simulink library "lib_wheel2"  (Simulink 4.1.1)
values from neighbouring files (symbols this model uses):
  logFlag = 1    [advSACompMaskInit.m]    (also in advSACompMaskInitR13.m)
undefined symbols (not defined in the file or in its folder): lib_help, NOTES, veh_air_density, veh_CD, veh_cg_height, veh_FA, veh_front_wt_frac, veh_gravity, veh_roadwheel_radius, veh_rr_a, veh_rr_alpha, veh_rr_b, veh_rr_beta, veh_rr_c, veh_wheelbase, wh_1st_rrc, wh_2nd_rrc, wh_axle_loss_mass, wh_axle_loss_trq, wh_fa_dl_brake_frac, wh_fa_dl_brake_mph, wh_fa_fric_brake_frac, wh_fa_fric_brake_mph, wh_front_active_bool, wh_inertia, wh_max_front_brake_force, wh_max_rear_brake_force, wh_pressure, wh_radius, wh_rear_active_bool, wh_slip, wh_slip_force_coeff
libraries: lib_wheel2 x61, lib_vehicle x2, lib_etc x2, lib_controls x2, lib_wheel x1
(part 10 of 14)

== system lib_wheel2/vehicle, wheel, & axle front/rear <wh>/models and interface/wheel and axle  front/rear <wh>/limits and losses diagnostics ==
  speed : Inport  Orientation=down  Port=1  LatchInput=off
  front brake : Inport  Port=2  LatchInput=off
  front brake max : Inport  Port=3  LatchInput=off
  rear brake max : Inport  Port=4  LatchInput=off
  rear brake : Inport  Port=5  LatchInput=off
  Gain : Gain  Gain=-1  Multiplication=Element-wise(K.*u)  SaturateOnIntegerOverflow=on
  Logical Operator : Logic  Operator=OR  Inputs=2
  Product : Product  Inputs=2  Multiplication=Element-wise(.*)  SaturateOnIntegerOverflow=on
  Relational Operator1 : RelationalOperator  Operator===
  Relational Operator2 : RelationalOperator  Operator===
  Sum3 : Sum  Inputs=++  SaturateOnIntegerOverflow=on
  enhancedToWorkspace : Subsystem  TreatAsAtomicUnit=on  mask(enhancedToWorkspace){generalName=generalName01, specificName=brake_loss_pwr, logFlag=logFlag}
      mask prompts: generalName "General Name [char-evaluated]"; specificName "Specific Name [char-literal]"; logFlag "Enable flag (1=on,0=off)"
      mask help: A wrapper for the Simulink "To Workspace" block that allows you to evaluate the name of the variable to log to workspace. This is useful to avoid the double logging errors that occur when you pull in two library models that attempt to log to the same variable.
      mask init:
      | enhancedToWsMaker
      settings: CopyFcn=breakLinkCopyFcn  ParentCloseFcn=breakLinkParCloseFcn  RTWFcnNameOpts=Auto  RTWFileNameOpts=Auto
      mask Help:
      | <h2>Enhanced To Workspace Block</h2>
      | <h3>Parameters</h3>
      | <UL>
      | <li><b>General Name:</b> This is the more general name of the variable. Variables are saved to the workspace as <i>generalName_specificName</i>. Note that this is an evaluated variable. If you would like to type in the value directly, it must be surrounded with single quotes. Otherwise you can input the name of a variable containing a char string.</li>
      | <li><b>Specific Name:</b> This is the specific name of the variable. Note that this is input as a char literal (i.e., you don't need quotes).</li>
      | <li><b>Enable Flag:</b> This flag should have the value of 0 or 1. If 0, the variable will not be logged to the workspace. If 1, the variable will be logged. This is done so that variable logging can be turned off to improve speed.</li>
      | </ul>
      | <h3>Overview</h3>
      | <p>The enhanced to workspace block was put together to allow one to dynamically resolve variable names at run time in simulink. This is most powerful when used in conjunction with a masked subsystem to allow multiple instances of that masked subsytem to be used in the same model. The strategy is to set the generalName in the block mask which will allow the block to change the general name for all variable logging on the fly.
      | <h3>Helper Files</h3>
      | <p>Three m-files are required by the enhancedToWorkspace block. These files are located in the &lt; ADVISOR root &gt;/GUI directory :
      | <ul>
      | <li><i>enhancedToWsMaker.m</i> This file runs the mask initialization for the block</li>
      | <li><i>breakLinkCopyFcn.m</i> This file is used by the block callback when the simulink block is copied. It is necessary to break the link to the enhancedToWorkspace similar to the To Workspace block in order for it to be able to configure itself. (Try copying simulink's To Workspace block--it is impossible to make a link)</li>
      | <li><i>breakLinkParCloseFcn.m</i> This file is similar to the breakLinkCopyFcn and is used when a parent system is closed</li>
      | </ul>
      | <hr>
      | 
      | <p>Created 2003-Jan-21, Michael Patrick O'Keefe, NREL</p>
      | 
      | <!--
      | <VARDEF>
      | <H3>var_name</H3>
      | <UL>
      | <LI><B>data type</B> data type here</LI>
      | <LI><B>units</B> units here</LI>
      | <LI><B>vehicle type</B> vehicle type here</LI>
      | <LI><B>description</B> description here</LI>
      | </UL>
      | </VARDEF>
      | -->
      mask Display: disp([generalName,'_',specificName])
  tag scope: brake_limited=scoped
  wires:
  Gain/1 -> Product/2
  Sum3/1 -> Gain/1
  Product/1 -> enhancedToWorkspace/1(In1)
  Logical Operator/1 -> [brake_limited]
  Relational Operator1/1 -> Logical Operator/1
  Relational Operator2/1 -> Logical Operator/2
  speed/1 -> Product/1
  front brake/1 -> Sum3/1, Relational Operator1/1
  front brake max/1 -> Relational Operator1/2
  rear brake max/1 -> Relational Operator2/1
  rear brake/1 -> Sum3/2, Relational Operator2/2

== system lib_wheel2/vehicle, wheel, & axle front/rear <wh>/models and interface/wheel and axle  front/rear <wh>/loss (Nm) ==
  note: The loss torque is zero when the axle is not turning.
  axle speed (rad/s) : Inport  Port=1  LatchInput=off
  Constant : Constant  Orientation=up  Value=0
  Switch : Switch  Threshold=eps
  current veh mass : lib_wheel2/Submodels/current veh mass
      settings: RTWFcnNameOpts=Auto  RTWFileNameOpts=Auto
  wheel & axle bearing drag (Nm) : Lookup  InputValues=wh_axle_loss_mass  OutputValues=wh_axle_loss_trq
  drag torque (Nm) : Outport  Port=1  InitialOutput=0
  wires:
  current veh mass/1 -> wheel & axle bearing drag (Nm)/1
  Switch/1 -> drag torque (Nm)/1
  axle speed (rad/s)/1 -> Switch/2
  Constant/1 -> Switch/3
  wheel & axle bearing drag (Nm)/1 -> Switch/1

== system lib_wheel2/vehicle, wheel, & axle front/rear <wh>/models and interface/wheel and axle  front/rear <wh>/rear brake ==
  F_brake : Inport  Port=1  LatchInput=off
  Constant : Constant  Value=wh_max_rear_brake_force
  Terminator : Terminator
  F_brake_max : Outport  Port=1  InitialOutput=0
  wires:
  Constant/1 -> F_brake_max/1
  F_brake/1 -> Terminator/1

== system lib_wheel2/vehicle, wheel, & axle front/rear <wh>/models and interface/wheel and axle  front/rear <wh>/rear force ==
  In1 : Inport  Port=1  LatchInput=off
  In2 : Inport  Port=2  LatchInput=off
  Product2 : Product  Inputs=2  Multiplication=Element-wise(.*)  SaturateOnIntegerOverflow=on
  Sum1 : Sum  Inputs=-+  SaturateOnIntegerOverflow=on
  Sum4 : Sum  Inputs=-+  SaturateOnIntegerOverflow=on
  brake request controller interface1 : Subsystem
      settings: RTWFcnNameOpts=Auto  RTWFileNameOpts=Auto
  enhancedToWorkspace : Subsystem  TreatAsAtomicUnit=on  mask(enhancedToWorkspace){generalName=generalName01, specificName=rear_brake_r, logFlag=logFlag}
      mask prompts: generalName "General Name [char-evaluated]"; specificName "Specific Name [char-literal]"; logFlag "Enable flag (1=on,0=off)"
      mask help: A wrapper for the Simulink "To Workspace" block that allows you to evaluate the name of the variable to log to workspace. This is useful to avoid the double logging errors that occur when you pull in two library models that attempt to log to the same variable.
      mask init:
      | enhancedToWsMaker
      settings: CopyFcn=breakLinkCopyFcn  ParentCloseFcn=breakLinkParCloseFcn  RTWFcnNameOpts=Auto  RTWFileNameOpts=Auto
      mask Help:
      | <h2>Enhanced To Workspace Block</h2>
      | <h3>Parameters</h3>
      | <UL>
      | <li><b>General Name:</b> This is the more general name of the variable. Variables are saved to the workspace as <i>generalName_specificName</i>. Note that this is an evaluated variable. If you would like to type in the value directly, it must be surrounded with single quotes. Otherwise you can input the name of a variable containing a char string.</li>
      | <li><b>Specific Name:</b> This is the specific name of the variable. Note that this is input as a char literal (i.e., you don't need quotes).</li>
      | <li><b>Enable Flag:</b> This flag should have the value of 0 or 1. If 0, the variable will not be logged to the workspace. If 1, the variable will be logged. This is done so that variable logging can be turned off to improve speed.</li>
      | </ul>
      | <h3>Overview</h3>
      | <p>The enhanced to workspace block was put together to allow one to dynamically resolve variable names at run time in simulink. This is most powerful when used in conjunction with a masked subsystem to allow multiple instances of that masked subsytem to be used in the same model. The strategy is to set the generalName in the block mask which will allow the block to change the general name for all variable logging on the fly.
      | <h3>Helper Files</h3>
      | <p>Three m-files are required by the enhancedToWorkspace block. These files are located in the &lt; ADVISOR root &gt;/GUI directory :
      | <ul>
      | <li><i>enhancedToWsMaker.m</i> This file runs the mask initialization for the block</li>
      | <li><i>breakLinkCopyFcn.m</i> This file is used by the block callback when the simulink block is copied. It is necessary to break the link to the enhancedToWorkspace similar to the To Workspace block in order for it to be able to configure itself. (Try copying simulink's To Workspace block--it is impossible to make a link)</li>
      | <li><i>breakLinkParCloseFcn.m</i> This file is similar to the breakLinkCopyFcn and is used when a parent system is closed</li>
      | </ul>
      | <hr>
      | 
      | <p>Created 2003-Jan-21, Michael Patrick O'Keefe, NREL</p>
      | 
      | <!--
      | <VARDEF>
      | <H3>var_name</H3>
      | <UL>
      | <LI><B>data type</B> data type here</LI>
      | <LI><B>units</B> units here</LI>
      | <LI><B>vehicle type</B> vehicle type here</LI>
      | <LI><B>description</B> description here</LI>
      | </UL>
      | </VARDEF>
      | -->
      mask Display: disp([generalName,'_',specificName])
  tractive torque req/d of drivetrain (Nm)1 : Gain  Gain=wh_radius  Multiplication=Element-wise(K.*u)  SaturateOnIntegerOverflow=on
  Out1 : Outport  Port=1
  wires:
  brake request controller interface1/1(F_rear_brake_req) -> Sum4/1, enhancedToWorkspace/1(In1)
  Sum4/1 -> tractive torque req/d of drivetrain (Nm)1/1
  tractive torque req/d of drivetrain (Nm)1/1 -> Out1/1
  In1/1 -> Product2/1, Sum1/2
  In2/1 -> Product2/2
  Product2/1 -> Sum1/1
  Sum1/1 -> Sum4/2

== system lib_wheel2/vehicle, wheel, & axle front/rear <wh>/models and interface/wheel and axle  front/rear <wh>/tire slip model (m/s) ==
  note: See note regarding sum in backward path
  weight borne  by front axle (N) : Inport  Port=1  LatchInput=off
  total tractive  force available (N) : Inport  Port=2  LatchInput=off
  axle speed available (rad/s) : Inport  Port=3  LatchInput=off
  axle speed req'd (rad/s) : Inport  Port=4  LatchInput=off
  vehicle speed required (m/s) : Inport  Port=5  LatchInput=off
  weight borne by  rear axle (N) : Inport  Port=6  LatchInput=off
  front fraction : Inport  Port=7  LatchInput=off
  Abs1 : Abs  SaturateOnIntegerOverflow=on
  Block NOTES : Subsystem
      settings: RTWFcnNameOpts=Auto  RTWFileNameOpts=Auto
      mask Display: disp('Block\nNOTES')
  Constant : Constant  Orientation=left  Value=1e-3
  Constant5 : Constant  Value=1
  Constant6 : Constant  Orientation=left  Value=wh_radius
  Fcn : Fcn  Expr=1/u
  Relational Operator1 : RelationalOperator  Operator=>
  Sum1 : Sum  Inputs=+-  SaturateOnIntegerOverflow=on
  Sum2 : Sum  Inputs=++  SaturateOnIntegerOverflow=on
  Sum3 : Sum  Inputs=++  SaturateOnIntegerOverflow=on
  Sum4 : Sum  Inputs=-+  SaturateOnIntegerOverflow=on
  Switch1 : Switch  Threshold=eps
  front axle : Subsystem
      settings: RTWFcnNameOpts=Auto  RTWFileNameOpts=Auto
  front frac : Product  Inputs=2  Multiplication=Element-wise(.*)  SaturateOnIntegerOverflow=on
  rear axle : Subsystem
      settings: RTWFcnNameOpts=Auto  RTWFileNameOpts=Auto
  vehicle speed (m/s) : Product  Inputs=3  Multiplication=Element-wise(.*)  SaturateOnIntegerOverflow=on
  possible vehicle speed (m/s) : Outport  Port=1  InitialOutput=0
  tag scope: veh_spd_a_rec=scoped
  wires:
  Sum3/1 -> Fcn/1
  Fcn/1 -> vehicle speed (m/s)/1
  Constant5/1 -> Sum3/2
  axle speed available (rad/s)/1 -> Sum4/1, vehicle speed (m/s)/2
  Constant6/1 -> vehicle speed (m/s)/3
  Relational Operator1/1 -> Switch1/2
  vehicle speed required (m/s)/1 -> Switch1/3
  Sum4/1 -> Abs1/1
  axle speed req'd (rad/s)/1 -> Sum4/2
  Constant/1 -> Relational Operator1/2
  Abs1/1 -> Relational Operator1/1
  weight borne  by front axle (N)/1 -> front axle/1(In1)
  Switch1/1 -> possible vehicle speed (m/s)/1
  vehicle speed (m/s)/1 -> Switch1/1, [veh_spd_a_rec]
  weight borne by  rear axle (N)/1 -> rear axle/1(In1)
  total tractive  force available (N)/1 -> front frac/1, Sum1/1
  front fraction/1 -> front frac/2
  front frac/1 -> front axle/2(In2), Sum1/2
  Sum1/1 -> rear axle/2(In2)
  front axle/1(Out1) -> Sum2/1
  rear axle/1(Out1) -> Sum2/2
  Sum2/1 -> Sum3/1

== system lib_wheel2/vehicle, wheel, & axle front/rear <wh>/models and interface/wheel and axle  front/rear <wh>/tire slip model (rad/s) ==
  note: Slip is defined as s=(omega*r - v) / v.  The one-to-one mapping of slip to normalized
      | tractive force, F_tract/W_front_axle, up to the maximum, is stored in the variables
      | "wh_slip" and "wh_slip_force_coeff."
  note: This block implements the effects of finite tire slip
      | (with respect to the road) on the vehicle speed/wheel speed relationship.
  note: Question: for front and rear, is it the sum of or min/max? tm:020703
  total tractive  force requested (N) : Inport  Port=1  LatchInput=off
  requested time-step average vehicle speed (m/s) : Inport  Port=2  LatchInput=off
  weight borne by front axle (N) : Inport  Port=3  LatchInput=off
  weight borne by  rear axle (N)1 : Inport  Port=4  LatchInput=off
  front traction ratio : Inport  Port=5  LatchInput=off
  Constant5 : Constant  Value=1
  Constant6 : Constant  Orientation=up  Value=1/wh_radius
  Sum1 : Sum  Inputs=+-  SaturateOnIntegerOverflow=on
  Sum2 : Sum  Inputs=++  SaturateOnIntegerOverflow=on
  Sum3 : Sum  Inputs=++  SaturateOnIntegerOverflow=on
  enhancedToWorkspace : Subsystem  TreatAsAtomicUnit=on  mask(enhancedToWorkspace){generalName=generalName01, specificName=slip_r, logFlag=logFlag}
      mask prompts: generalName "General Name [char-evaluated]"; specificName "Specific Name [char-literal]"; logFlag "Enable flag (1=on,0=off)"
      mask help: A wrapper for the Simulink "To Workspace" block that allows you to evaluate the name of the variable to log to workspace. This is useful to avoid the double logging errors that occur when you pull in two library models that attempt to log to the same variable.
      mask init:
      | enhancedToWsMaker
      settings: CopyFcn=breakLinkCopyFcn  ParentCloseFcn=breakLinkParCloseFcn  RTWFcnNameOpts=Auto  RTWFileNameOpts=Auto
      mask Help:
      | <h2>Enhanced To Workspace Block</h2>
      | <h3>Parameters</h3>
      | <UL>
      | <li><b>General Name:</b> This is the more general name of the variable. Variables are saved to the workspace as <i>generalName_specificName</i>. Note that this is an evaluated variable. If you would like to type in the value directly, it must be surrounded with single quotes. Otherwise you can input the name of a variable containing a char string.</li>
      | <li><b>Specific Name:</b> This is the specific name of the variable. Note that this is input as a char literal (i.e., you don't need quotes).</li>
      | <li><b>Enable Flag:</b> This flag should have the value of 0 or 1. If 0, the variable will not be logged to the workspace. If 1, the variable will be logged. This is done so that variable logging can be turned off to improve speed.</li>
      | </ul>
      | <h3>Overview</h3>
      | <p>The enhanced to workspace block was put together to allow one to dynamically resolve variable names at run time in simulink. This is most powerful when used in conjunction with a masked subsystem to allow multiple instances of that masked subsytem to be used in the same model. The strategy is to set the generalName in the block mask which will allow the block to change the general name for all variable logging on the fly.
      | <h3>Helper Files</h3>
      | <p>Three m-files are required by the enhancedToWorkspace block. These files are located in the &lt; ADVISOR root &gt;/GUI directory :
      | <ul>
      | <li><i>enhancedToWsMaker.m</i> This file runs the mask initialization for the block</li>
      | <li><i>breakLinkCopyFcn.m</i> This file is used by the block callback when the simulink block is copied. It is necessary to break the link to the enhancedToWorkspace similar to the To Workspace block in order for it to be able to configure itself. (Try copying simulink's To Workspace block--it is impossible to make a link)</li>
      | <li><i>breakLinkParCloseFcn.m</i> This file is similar to the breakLinkCopyFcn and is used when a parent system is closed</li>
      | </ul>
      | <hr>
      | 
      | <p>Created 2003-Jan-21, Michael Patrick O'Keefe, NREL</p>
      | 
      | <!--
      | <VARDEF>
      | <H3>var_name</H3>
      | <UL>
      | <LI><B>data type</B> data type here</LI>
      | <LI><B>units</B> units here</LI>
      | <LI><B>vehicle type</B> vehicle type here</LI>
      | <LI><B>description</B> description here</LI>
      | </UL>
      | </VARDEF>
      | -->
      mask Display: disp([generalName,'_',specificName])
  front frac : Product  Inputs=2  Multiplication=Element-wise(.*)  SaturateOnIntegerOverflow=on
  front slip : Subsystem
      settings: RTWFcnNameOpts=Auto  RTWFileNameOpts=Auto
  rear slip : Subsystem
      settings: RTWFcnNameOpts=Auto  RTWFileNameOpts=Auto
  wheel speed (rad/s) : Product  Inputs=3  Multiplication=Element-wise(.*)  SaturateOnIntegerOverflow=on
  slip-augmented rotational speed (rad/s) : Outport  Port=1  InitialOutput=0
  wires:
  weight borne by front axle (N)/1 -> front slip/1(In1)
  requested time-step average vehicle speed (m/s)/1 -> wheel speed (rad/s)/1
  Constant6/1 -> wheel speed (rad/s)/3
  Sum3/1 -> wheel speed (rad/s)/2
  Constant5/1 -> Sum3/2
  wheel speed (rad/s)/1 -> slip-augmented rotational speed (rad/s)/1
  front frac/1 -> Sum1/2, front slip/2(In2)
  total tractive  force requested (N)/1 -> front frac/1, Sum1/1
  front traction ratio/1 -> front frac/2
  Sum1/1 -> rear slip/2(In2)
  weight borne by  rear axle (N)1/1 -> rear slip/1(In1)
  front slip/1(Out1) -> Sum2/1
  rear slip/1(Out1) -> Sum2/2
  Sum2/1 -> Sum3/1, enhancedToWorkspace/1(In1)

== system lib_wheel2/vehicle, wheel, & axle front/rear <wh>/models and interface/wheel and axle  front/rear <wh>/traction controller interface ==
  F_req : Inport  Port=1  LatchInput=off
  v_ave_req : Inport  Port=2  LatchInput=off
  F_req_limited : Outport  Port=1  InitialOutput=0
  v_req_limited : Outport  Port=2  InitialOutput=0
  wt_front_axle : Outport  Port=3  InitialOutput=0
  wt_rear_axle : Outport  Port=4  InitialOutput=0
  front_traction_ratio : Outport  Port=5  InitialOutput=0
  tag scope: F_req=scoped, v_ave_req=scoped
  wires:
  [F_req_limited] -> F_req_limited/1
  [v_req_limited] -> v_req_limited/1
  [wt_front_axle] -> wt_front_axle/1
  F_req/1 -> [F_req]
  v_ave_req/1 -> [v_ave_req]
  [wt_rear_axle] -> wt_rear_axle/1
  [front_traction_ratio] -> front_traction_ratio/1

== system lib_wheel2/vehicle, wheel, & axle front/rear <wh> 2 axle --> 1 driveline/models and interface/vehicle <veh>/Block NOTES ==
  note: Given the tractive force available, this block uses the same equations to determine the achievable speed.
  note: If no drivetrain component ran up against its performance limit during the time step, the achieved speed
      | is taken to be the requested speed.
  note: This block uses the required vehicle speed with vehicle parameters and the previous speed
      | and classic, straightforward equations to determine the tractive force required at the tire/road interface.
  note: A slight simplification, the assumption that (speed_at_end_of_time_step)^2 is roughly equal to
      | (speed_at_end_of_time_step)*(speed_at_beginning_of_time_step), is used to avoid solving
      | a quadratic equation in the solution of v=v(Ftract).
  note: 2003-April-02, Michael O'Keefe
      | Model updated to use a "stand-alone" mask format

== system lib_wheel2/vehicle, wheel, & axle front/rear <wh> 2 axle --> 1 driveline/models and interface/vehicle <veh>/enhancedToWorkspace ==
  In1 : Inport  Port=1  LatchInput=off
  To Workspace : ToWorkspace  VariableName=veh_spd_a  SampleTime=-1  SaveFormat=Array
  wires:
  In1/1 -> To Workspace/1

== system lib_wheel2/vehicle, wheel, & axle front/rear <wh> 2 axle --> 1 driveline/models and interface/vehicle <veh>/enhancedToWorkspace1 ==
  In1 : Inport  Port=1  LatchInput=off
  To Workspace : ToWorkspace  VariableName=veh_force_a  SampleTime=-1  SaveFormat=Array
  wires:
  In1/1 -> To Workspace/1

== system lib_wheel2/vehicle, wheel, & axle front/rear <wh> 2 axle --> 1 driveline/models and interface/vehicle <veh>/enhancedToWorkspace2 ==
  In1 : Inport  Port=1  LatchInput=off
  To Workspace : ToWorkspace  VariableName=veh_spd_r  SampleTime=-1  SaveFormat=Array
  wires:
  In1/1 -> To Workspace/1

== system lib_wheel2/vehicle, wheel, & axle front/rear <wh> 2 axle --> 1 driveline/models and interface/vehicle <veh>/enhancedToWorkspace3 ==
  In1 : Inport  Port=1  LatchInput=off
  To Workspace : ToWorkspace  VariableName=veh_force_r  SampleTime=-1  SaveFormat=Array
  wires:
  In1/1 -> To Workspace/1

== system lib_wheel2/vehicle, wheel, & axle front/rear <wh> 2 axle --> 1 driveline/models and interface/vehicle <veh>/enhancedToWorkspace4 ==
  In1 : Inport  Port=1  LatchInput=off
  To Workspace : ToWorkspace  VariableName=veh_Fr  SampleTime=-1  SaveFormat=Array
  wires:
  In1/1 -> To Workspace/1

== system lib_wheel2/vehicle, wheel, & axle front/rear <wh> 2 axle --> 1 driveline/models and interface/vehicle <veh>/force req'd to accelerate (N) ==
  v(m/s) : Inport  Port=1  LatchInput=off
  v prev : Inport  Port=2  LatchInput=off
  Clock : Clock
      settings: DisplayTime=off  Decimation=10
  Memory : Memory  X0=-0.1  InheritSampleTime=off
      settings: RTWStateStorageClass=Auto
  Product1 : Product  Inputs=**/  Multiplication=Element-wise(.*)  SaturateOnIntegerOverflow=on
  Sum : Sum  Inputs=+-  SaturateOnIntegerOverflow=on
  Sum1 : Sum  Inputs=+-  SaturateOnIntegerOverflow=on
  current veh mass : lib_wheel2/Submodels/current veh mass
      settings: RTWFcnNameOpts=Auto  RTWFileNameOpts=Auto
  (N) : Outport  Port=1  InitialOutput=0
  wires:
  Sum/1 -> Product1/2
  Sum1/1 -> Product1/3
  v(m/s)/1 -> Sum/1
  v prev/1 -> Sum/2
  Product1/1 -> (N)/1
  Memory/1 -> Sum1/2
  Clock/1 -> Memory/1, Sum1/1
  current veh mass/1 -> Product1/1

== system lib_wheel2/vehicle, wheel, & axle front/rear <wh> 2 axle --> 1 driveline/models and interface/vehicle <veh>/force req'd to ascend (N) ==
  average vehicle speed over time step (m/s) : Inport  Port=1  LatchInput=off
  Constant : Constant  Value=veh_gravity
  Constant1 : Constant  Value=0
  Product : Product  Inputs=3  Multiplication=Element-wise(.*)  SaturateOnIntegerOverflow=on
  Switch : Switch  Threshold=0
  Trigonometric Function : Trigonometry  Operator=atan  OutputSignalType=auto
  Trigonometric Function1 : Trigonometry  Operator=sin  OutputSignalType=auto
  current veh mass : lib_wheel2/Submodels/current veh mass
      settings: RTWFcnNameOpts=Auto  RTWFileNameOpts=Auto
  (N) : Outport  Port=1  InitialOutput=0
  wires:
  Trigonometric Function/1 -> Trigonometric Function1/1
  Trigonometric Function1/1 -> Product/2
  [grade] -> Trigonometric Function/1
  Constant/1 -> Product/1
  Product/1 -> Switch/1
  Switch/1 -> (N)/1
  Constant1/1 -> Switch/3
  average vehicle speed over time step (m/s)/1 -> Switch/2
  current veh mass/1 -> Product/3

== system lib_wheel2/vehicle, wheel, & axle front/rear <wh> 2 axle --> 1 driveline/models and interface/vehicle <veh>/force req'd to overcome aerodynamic drag (N) ==
  average vehicle speed over time step (m/s) : Inport  Port=1  LatchInput=off
  Constant : Constant  Value=veh_air_density*veh_CD*veh_FA*0.5
  Product : Product  Inputs=3  Multiplication=Element-wise(.*)  SaturateOnIntegerOverflow=on
  D aero(N) : Outport  Port=1  InitialOutput=0
  wires:
  average vehicle speed over time step (m/s)/1 -> Product/1, Product/2
  Constant/1 -> Product/3
  Product/1 -> D aero(N)/1

== system lib_wheel2/vehicle, wheel, & axle front/rear <wh> 2 axle --> 1 driveline/models and interface/vehicle <veh>/help ==

== system lib_wheel2/vehicle, wheel, & axle front/rear <wh> 2 axle --> 1 driveline/models and interface/vehicle <veh>/memory & init speed ==
  note: cyc_mph(1,2)*.447
  note: 2003-April-02, Michael O'Keefe
      |
      | This block passes through the last speed achieved unless this is the initial condition in which
      | case the initial speed value (a supplied control signal) is passed through. For backwards
      | compatibility, the value of v_init should be cyc_mph(1,2)*0.447
  signal in : Inport  Port=1  LatchInput=off
  signal init : Inport  Port=2  LatchInput=off
  Constant : Constant  Value=1
  IC : InitialCondition  Value=0
  Memory : Memory  X0=0  InheritSampleTime=off
      settings: RTWStateStorageClass=Auto
  Switch : Switch  Threshold=0.5
  signal out : Outport  Port=1
  wires:
  signal in/1 -> Memory/1
  Constant/1 -> IC/1
  Memory/1 -> Switch/1
  IC/1 -> Switch/2
  Switch/1 -> signal out/1
  signal init/1 -> Switch/3

== system lib_wheel2/vehicle, wheel, & axle front/rear <wh> 2 axle --> 1 driveline/models and interface/vehicle <veh>/power logging--achieved ==
  veh_force_a : Inport  Port=1  LatchInput=off
  veh_spd_a : Inport  Port=2  LatchInput=off
  Integrator : Integrator  ExternalReset=none  InitialConditionSource=internal  InitialCondition=0  LimitOutput=off  UpperSaturationLimit=inf  LowerSaturationLimit=-inf  ShowSaturationPort=off  ShowStatePort=off  AbsoluteTolerance=auto
  Joules : Subsystem  TreatAsAtomicUnit=on  mask(enhancedToWorkspace){generalName=generalName, specificName=energy_a, logFlag=logFlag}
      mask prompts: generalName "General Name [char-evaluated]"; specificName "Specific Name [char-literal]"; logFlag "Enable flag (1=on,0=off)"
      mask help: A wrapper for the Simulink "To Workspace" block that allows you to evaluate the name of the variable to log to workspace. This is useful to avoid the double logging errors that occur when you pull in two library models that attempt to log to the same variable.
      mask init:
      | enhancedToWsMaker
      settings: CopyFcn=breakLinkCopyFcn  ParentCloseFcn=breakLinkParCloseFcn  RTWFcnNameOpts=Auto  RTWFileNameOpts=Auto
      mask Help:
      | <h2>Enhanced To Workspace Block</h2>
      | <h3>Parameters</h3>
      | <UL>
      | <li><b>General Name:</b> This is the more general name of the variable. Variables are saved to the workspace as <i>generalName_specificName</i>. Note that this is an evaluated variable. If you would like to type in the value directly, it must be surrounded with single quotes. Otherwise you can input the name of a variable containing a char string.</li>
      | <li><b>Specific Name:</b> This is the specific name of the variable. Note that this is input as a char literal (i.e., you don't need quotes).</li>
      | <li><b>Enable Flag:</b> This flag should have the value of 0 or 1. If 0, the variable will not be logged to the workspace. If 1, the variable will be logged. This is done so that variable logging can be turned off to improve speed.</li>
      | </ul>
      | <h3>Overview</h3>
      | <p>The enhanced to workspace block was put together to allow one to dynamically resolve variable names at run time in simulink. This is most powerful when used in conjunction with a masked subsystem to allow multiple instances of that masked subsytem to be used in the same model. The strategy is to set the generalName in the block mask which will allow the block to change the general name for all variable logging on the fly.
      | <h3>Helper Files</h3>
      | <p>Three m-files are required by the enhancedToWorkspace block. These files are located in the &lt; ADVISOR root &gt;/GUI directory :
      | <ul>
      | <li><i>enhancedToWsMaker.m</i> This file runs the mask initialization for the block</li>
      | <li><i>breakLinkCopyFcn.m</i> This file is used by the block callback when the simulink block is copied. It is necessary to break the link to the enhancedToWorkspace similar to the To Workspace block in order for it to be able to configure itself. (Try copying simulink's To Workspace block--it is impossible to make a link)</li>
      | <li><i>breakLinkParCloseFcn.m</i> This file is similar to the breakLinkCopyFcn and is used when a parent system is closed</li>
      | </ul>
      | <hr>
      | 
      | <p>Created 2003-Jan-21, Michael Patrick O'Keefe, NREL</p>
      | 
      | <!--
      | <VARDEF>
      | <H3>var_name</H3>
      | <UL>
      | <LI><B>data type</B> data type here</LI>
      | <LI><B>units</B> units here</LI>
      | <LI><B>vehicle type</B> vehicle type here</LI>
      | <LI><B>description</B> description here</LI>
      | </UL>
      | </VARDEF>
      | -->
      mask Display: disp([generalName,'_',specificName])
  Product : Product  Inputs=2  Multiplication=Element-wise(.*)  SaturateOnIntegerOverflow=on
  horse power : Subsystem  TreatAsAtomicUnit=on  mask(enhancedToWorkspace){generalName=generalName, specificName=pwr_a_hp, logFlag=logFlag}
      mask prompts: generalName "General Name [char-evaluated]"; specificName "Specific Name [char-literal]"; logFlag "Enable flag (1=on,0=off)"
      mask help: A wrapper for the Simulink "To Workspace" block that allows you to evaluate the name of the variable to log to workspace. This is useful to avoid the double logging errors that occur when you pull in two library models that attempt to log to the same variable.
      mask init:
      | enhancedToWsMaker
      settings: CopyFcn=breakLinkCopyFcn  ParentCloseFcn=breakLinkParCloseFcn  RTWFcnNameOpts=Auto  RTWFileNameOpts=Auto
      mask Help:
      | <h2>Enhanced To Workspace Block</h2>
      | <h3>Parameters</h3>
      | <UL>
      | <li><b>General Name:</b> This is the more general name of the variable. Variables are saved to the workspace as <i>generalName_specificName</i>. Note that this is an evaluated variable. If you would like to type in the value directly, it must be surrounded with single quotes. Otherwise you can input the name of a variable containing a char string.</li>
      | <li><b>Specific Name:</b> This is the specific name of the variable. Note that this is input as a char literal (i.e., you don't need quotes).</li>
      | <li><b>Enable Flag:</b> This flag should have the value of 0 or 1. If 0, the variable will not be logged to the workspace. If 1, the variable will be logged. This is done so that variable logging can be turned off to improve speed.</li>
      | </ul>
      | <h3>Overview</h3>
      | <p>The enhanced to workspace block was put together to allow one to dynamically resolve variable names at run time in simulink. This is most powerful when used in conjunction with a masked subsystem to allow multiple instances of that masked subsytem to be used in the same model. The strategy is to set the generalName in the block mask which will allow the block to change the general name for all variable logging on the fly.
      | <h3>Helper Files</h3>
      | <p>Three m-files are required by the enhancedToWorkspace block. These files are located in the &lt; ADVISOR root &gt;/GUI directory :
      | <ul>
      | <li><i>enhancedToWsMaker.m</i> This file runs the mask initialization for the block</li>
      | <li><i>breakLinkCopyFcn.m</i> This file is used by the block callback when the simulink block is copied. It is necessary to break the link to the enhancedToWorkspace similar to the To Workspace block in order for it to be able to configure itself. (Try copying simulink's To Workspace block--it is impossible to make a link)</li>
      | <li><i>breakLinkParCloseFcn.m</i> This file is similar to the breakLinkCopyFcn and is used when a parent system is closed</li>
      | </ul>
      | <hr>
      | 
      | <p>Created 2003-Jan-21, Michael Patrick O'Keefe, NREL</p>
      | 
      | <!--
      | <VARDEF>
      | <H3>var_name</H3>
      | <UL>
      | <LI><B>data type</B> data type here</LI>
      | <LI><B>units</B> units here</LI>
      | <LI><B>vehicle type</B> vehicle type here</LI>
      | <LI><B>description</B> description here</LI>
      | </UL>
      | </VARDEF>
      | -->
      mask Display: disp([generalName,'_',specificName])
  "w -> hp" : Gain  Gain=0.001341022  Multiplication=Element-wise(K.*u)  SaturateOnIntegerOverflow=on
  watts : Subsystem  TreatAsAtomicUnit=on  mask(enhancedToWorkspace){generalName=generalName, specificName=pwr_a, logFlag=logFlag}
      mask prompts: generalName "General Name [char-evaluated]"; specificName "Specific Name [char-literal]"; logFlag "Enable flag (1=on,0=off)"
      mask help: A wrapper for the Simulink "To Workspace" block that allows you to evaluate the name of the variable to log to workspace. This is useful to avoid the double logging errors that occur when you pull in two library models that attempt to log to the same variable.
      mask init:
      | enhancedToWsMaker
      settings: CopyFcn=breakLinkCopyFcn  ParentCloseFcn=breakLinkParCloseFcn  RTWFcnNameOpts=Auto  RTWFileNameOpts=Auto
      mask Help:
      | <h2>Enhanced To Workspace Block</h2>
      | <h3>Parameters</h3>
      | <UL>
      | <li><b>General Name:</b> This is the more general name of the variable. Variables are saved to the workspace as <i>generalName_specificName</i>. Note that this is an evaluated variable. If you would like to type in the value directly, it must be surrounded with single quotes. Otherwise you can input the name of a variable containing a char string.</li>
      | <li><b>Specific Name:</b> This is the specific name of the variable. Note that this is input as a char literal (i.e., you don't need quotes).</li>
      | <li><b>Enable Flag:</b> This flag should have the value of 0 or 1. If 0, the variable will not be logged to the workspace. If 1, the variable will be logged. This is done so that variable logging can be turned off to improve speed.</li>
      | </ul>
      | <h3>Overview</h3>
      | <p>The enhanced to workspace block was put together to allow one to dynamically resolve variable names at run time in simulink. This is most powerful when used in conjunction with a masked subsystem to allow multiple instances of that masked subsytem to be used in the same model. The strategy is to set the generalName in the block mask which will allow the block to change the general name for all variable logging on the fly.
      | <h3>Helper Files</h3>
      | <p>Three m-files are required by the enhancedToWorkspace block. These files are located in the &lt; ADVISOR root &gt;/GUI directory :
      | <ul>
      | <li><i>enhancedToWsMaker.m</i> This file runs the mask initialization for the block</li>
      | <li><i>breakLinkCopyFcn.m</i> This file is used by the block callback when the simulink block is copied. It is necessary to break the link to the enhancedToWorkspace similar to the To Workspace block in order for it to be able to configure itself. (Try copying simulink's To Workspace block--it is impossible to make a link)</li>
      | <li><i>breakLinkParCloseFcn.m</i> This file is similar to the breakLinkCopyFcn and is used when a parent system is closed</li>
      | </ul>
      | <hr>
      | 
      | <p>Created 2003-Jan-21, Michael Patrick O'Keefe, NREL</p>
      | 
      | <!--
      | <VARDEF>
      | <H3>var_name</H3>
      | <UL>
      | <LI><B>data type</B> data type here</LI>
      | <LI><B>units</B> units here</LI>
      | <LI><B>vehicle type</B> vehicle type here</LI>
      | <LI><B>description</B> description here</LI>
      | </UL>
      | </VARDEF>
      | -->
      mask Display: disp([generalName,'_',specificName])
  wires:
  veh_spd_a/1 -> Product/2
  veh_force_a/1 -> Product/1
  Integrator/1 -> Joules/1(In1)
  Product/1 -> watts/1(In1), Integrator/1, "w -> hp"/1
  "w -> hp"/1 -> horse power/1(In1)

== system lib_wheel2/vehicle, wheel, & axle front/rear <wh> 2 axle --> 1 driveline/models and interface/vehicle <veh>/power logging--request ==
  veh_force_r : Inport  Port=1  LatchInput=off
  veh_spd_r : Inport  Port=2  LatchInput=off
  Integrator : Integrator  ExternalReset=none  InitialConditionSource=internal  InitialCondition=0  LimitOutput=off  UpperSaturationLimit=inf  LowerSaturationLimit=-inf  ShowSaturationPort=off  ShowStatePort=off  AbsoluteTolerance=auto
  Joules : Subsystem  TreatAsAtomicUnit=on  mask(enhancedToWorkspace){generalName=generalName, specificName=energy_r, logFlag=logFlag}
      mask prompts: generalName "General Name [char-evaluated]"; specificName "Specific Name [char-literal]"; logFlag "Enable flag (1=on,0=off)"
      mask help: A wrapper for the Simulink "To Workspace" block that allows you to evaluate the name of the variable to log to workspace. This is useful to avoid the double logging errors that occur when you pull in two library models that attempt to log to the same variable.
      mask init:
      | enhancedToWsMaker
      settings: CopyFcn=breakLinkCopyFcn  ParentCloseFcn=breakLinkParCloseFcn  RTWFcnNameOpts=Auto  RTWFileNameOpts=Auto
      mask Help:
      | <h2>Enhanced To Workspace Block</h2>
      | <h3>Parameters</h3>
      | <UL>
      | <li><b>General Name:</b> This is the more general name of the variable. Variables are saved to the workspace as <i>generalName_specificName</i>. Note that this is an evaluated variable. If you would like to type in the value directly, it must be surrounded with single quotes. Otherwise you can input the name of a variable containing a char string.</li>
      | <li><b>Specific Name:</b> This is the specific name of the variable. Note that this is input as a char literal (i.e., you don't need quotes).</li>
      | <li><b>Enable Flag:</b> This flag should have the value of 0 or 1. If 0, the variable will not be logged to the workspace. If 1, the variable will be logged. This is done so that variable logging can be turned off to improve speed.</li>
      | </ul>
      | <h3>Overview</h3>
      | <p>The enhanced to workspace block was put together to allow one to dynamically resolve variable names at run time in simulink. This is most powerful when used in conjunction with a masked subsystem to allow multiple instances of that masked subsytem to be used in the same model. The strategy is to set the generalName in the block mask which will allow the block to change the general name for all variable logging on the fly.
      | <h3>Helper Files</h3>
      | <p>Three m-files are required by the enhancedToWorkspace block. These files are located in the &lt; ADVISOR root &gt;/GUI directory :
      | <ul>
      | <li><i>enhancedToWsMaker.m</i> This file runs the mask initialization for the block</li>
      | <li><i>breakLinkCopyFcn.m</i> This file is used by the block callback when the simulink block is copied. It is necessary to break the link to the enhancedToWorkspace similar to the To Workspace block in order for it to be able to configure itself. (Try copying simulink's To Workspace block--it is impossible to make a link)</li>
      | <li><i>breakLinkParCloseFcn.m</i> This file is similar to the breakLinkCopyFcn and is used when a parent system is closed</li>
      | </ul>
      | <hr>
      | 
      | <p>Created 2003-Jan-21, Michael Patrick O'Keefe, NREL</p>
      | 
      | <!--
      | <VARDEF>
      | <H3>var_name</H3>
      | <UL>
      | <LI><B>data type</B> data type here</LI>
      | <LI><B>units</B> units here</LI>
      | <LI><B>vehicle type</B> vehicle type here</LI>
      | <LI><B>description</B> description here</LI>
      | </UL>
      | </VARDEF>
      | -->
      mask Display: disp([generalName,'_',specificName])
  Product : Product  Inputs=2  Multiplication=Element-wise(.*)  SaturateOnIntegerOverflow=on
  horse power : Subsystem  TreatAsAtomicUnit=on  mask(enhancedToWorkspace){generalName=generalName, specificName=pwr_r_hp, logFlag=logFlag}
      mask prompts: generalName "General Name [char-evaluated]"; specificName "Specific Name [char-literal]"; logFlag "Enable flag (1=on,0=off)"
      mask help: A wrapper for the Simulink "To Workspace" block that allows you to evaluate the name of the variable to log to workspace. This is useful to avoid the double logging errors that occur when you pull in two library models that attempt to log to the same variable.
      mask init:
      | enhancedToWsMaker
      settings: CopyFcn=breakLinkCopyFcn  ParentCloseFcn=breakLinkParCloseFcn  RTWFcnNameOpts=Auto  RTWFileNameOpts=Auto
      mask Help:
      | <h2>Enhanced To Workspace Block</h2>
      | <h3>Parameters</h3>
      | <UL>
      | <li><b>General Name:</b> This is the more general name of the variable. Variables are saved to the workspace as <i>generalName_specificName</i>. Note that this is an evaluated variable. If you would like to type in the value directly, it must be surrounded with single quotes. Otherwise you can input the name of a variable containing a char string.</li>
      | <li><b>Specific Name:</b> This is the specific name of the variable. Note that this is input as a char literal (i.e., you don't need quotes).</li>
      | <li><b>Enable Flag:</b> This flag should have the value of 0 or 1. If 0, the variable will not be logged to the workspace. If 1, the variable will be logged. This is done so that variable logging can be turned off to improve speed.</li>
      | </ul>
      | <h3>Overview</h3>
      | <p>The enhanced to workspace block was put together to allow one to dynamically resolve variable names at run time in simulink. This is most powerful when used in conjunction with a masked subsystem to allow multiple instances of that masked subsytem to be used in the same model. The strategy is to set the generalName in the block mask which will allow the block to change the general name for all variable logging on the fly.
      | <h3>Helper Files</h3>
      | <p>Three m-files are required by the enhancedToWorkspace block. These files are located in the &lt; ADVISOR root &gt;/GUI directory :
      | <ul>
      | <li><i>enhancedToWsMaker.m</i> This file runs the mask initialization for the block</li>
      | <li><i>breakLinkCopyFcn.m</i> This file is used by the block callback when the simulink block is copied. It is necessary to break the link to the enhancedToWorkspace similar to the To Workspace block in order for it to be able to configure itself. (Try copying simulink's To Workspace block--it is impossible to make a link)</li>
      | <li><i>breakLinkParCloseFcn.m</i> This file is similar to the breakLinkCopyFcn and is used when a parent system is closed</li>
      | </ul>
      | <hr>
      | 
      | <p>Created 2003-Jan-21, Michael Patrick O'Keefe, NREL</p>
      | 
      | <!--
      | <VARDEF>
      | <H3>var_name</H3>
      | <UL>
      | <LI><B>data type</B> data type here</LI>
      | <LI><B>units</B> units here</LI>
      | <LI><B>vehicle type</B> vehicle type here</LI>
      | <LI><B>description</B> description here</LI>
      | </UL>
      | </VARDEF>
      | -->
      mask Display: disp([generalName,'_',specificName])
  "w -> hp" : Gain  Gain=0.001341022  Multiplication=Element-wise(K.*u)  SaturateOnIntegerOverflow=on
  watts : Subsystem  TreatAsAtomicUnit=on  mask(enhancedToWorkspace){generalName=generalName, specificName=pwr_r, logFlag=logFlag}
      mask prompts: generalName "General Name [char-evaluated]"; specificName "Specific Name [char-literal]"; logFlag "Enable flag (1=on,0=off)"
      mask help: A wrapper for the Simulink "To Workspace" block that allows you to evaluate the name of the variable to log to workspace. This is useful to avoid the double logging errors that occur when you pull in two library models that attempt to log to the same variable.
      mask init:
      | enhancedToWsMaker
      settings: CopyFcn=breakLinkCopyFcn  ParentCloseFcn=breakLinkParCloseFcn  RTWFcnNameOpts=Auto  RTWFileNameOpts=Auto
      mask Help:
      | <h2>Enhanced To Workspace Block</h2>
      | <h3>Parameters</h3>
      | <UL>
      | <li><b>General Name:</b> This is the more general name of the variable. Variables are saved to the workspace as <i>generalName_specificName</i>. Note that this is an evaluated variable. If you would like to type in the value directly, it must be surrounded with single quotes. Otherwise you can input the name of a variable containing a char string.</li>
      | <li><b>Specific Name:</b> This is the specific name of the variable. Note that this is input as a char literal (i.e., you don't need quotes).</li>
      | <li><b>Enable Flag:</b> This flag should have the value of 0 or 1. If 0, the variable will not be logged to the workspace. If 1, the variable will be logged. This is done so that variable logging can be turned off to improve speed.</li>
      | </ul>
      | <h3>Overview</h3>
      | <p>The enhanced to workspace block was put together to allow one to dynamically resolve variable names at run time in simulink. This is most powerful when used in conjunction with a masked subsystem to allow multiple instances of that masked subsytem to be used in the same model. The strategy is to set the generalName in the block mask which will allow the block to change the general name for all variable logging on the fly.
      | <h3>Helper Files</h3>
      | <p>Three m-files are required by the enhancedToWorkspace block. These files are located in the &lt; ADVISOR root &gt;/GUI directory :
      | <ul>
      | <li><i>enhancedToWsMaker.m</i> This file runs the mask initialization for the block</li>
      | <li><i>breakLinkCopyFcn.m</i> This file is used by the block callback when the simulink block is copied. It is necessary to break the link to the enhancedToWorkspace similar to the To Workspace block in order for it to be able to configure itself. (Try copying simulink's To Workspace block--it is impossible to make a link)</li>
      | <li><i>breakLinkParCloseFcn.m</i> This file is similar to the breakLinkCopyFcn and is used when a parent system is closed</li>
      | </ul>
      | <hr>
      | 
      | <p>Created 2003-Jan-21, Michael Patrick O'Keefe, NREL</p>
      | 
      | <!--
      | <VARDEF>
      | <H3>var_name</H3>
      | <UL>
      | <LI><B>data type</B> data type here</LI>
      | <LI><B>units</B> units here</LI>
      | <LI><B>vehicle type</B> vehicle type here</LI>
      | <LI><B>description</B> description here</LI>
      | </UL>
      | </VARDEF>
      | -->
      mask Display: disp([generalName,'_',specificName])
  wires:
  veh_spd_r/1 -> Product/2
  veh_force_r/1 -> Product/1
  Integrator/1 -> Joules/1(In1)
  Product/1 -> watts/1(In1), Integrator/1, "w -> hp"/1
  "w -> hp"/1 -> horse power/1(In1)
